simulink model "esempio1S"  (R2021a)
settings: Solver=VariableStepAuto  StartTime=0.0  StopTime=10.0  RelTol=1e-3
values from neighbouring files (symbols this model uses):
  A = [0 1; 0 -2]    [esempio.m]    (also in esempio1.m = [-2 1; -2 0]; esempio2.m = [0 1; 2 1])
  B = [ 0; 1]    [esempio.m]    (also in esempio1.m = [0; 1]; esempio2.m = [0; 1])
  C = eye(2)    [esempio.m]    (also in esempio1.m; esempio2.m)
  D = zeros(2,1)    [esempio.m]    (also in esempio1.m; esempio2.m)
  K = place(A, B, P)    [esempio.m]    (also in esempio1.m = acker(A, B, P); esempio2.m)
  x0 = [0;0]    [esempio1.m]
settings Model: Creator=itama  LastModifiedBy=itama
settings SolverCC: AlgebraicLoopSolver=TrustRegion
settings DebuggingCC: SFMachineParentedDataDiag=warning

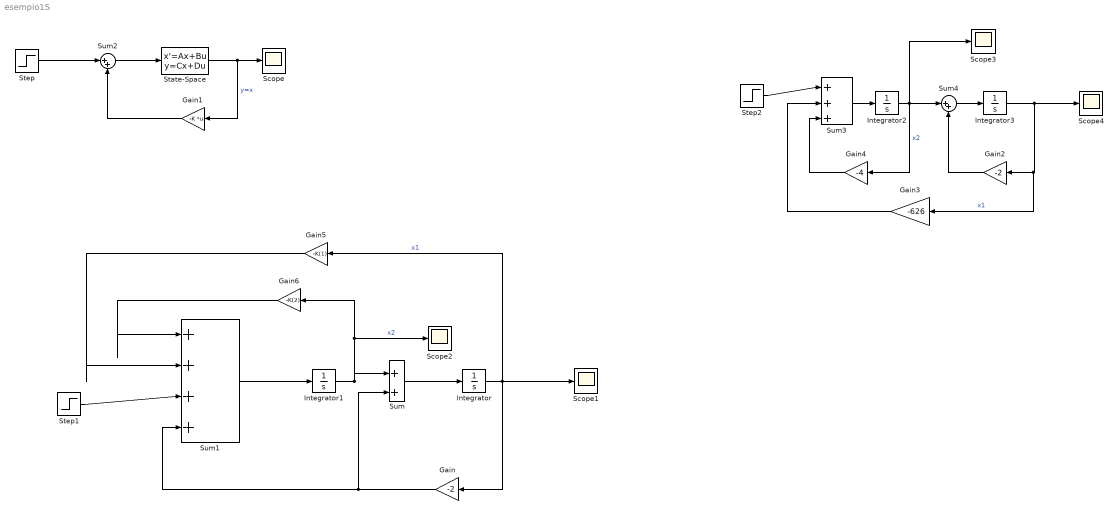
== system esempio1S ==
  Gain : Gain  Gain=-2
  Gain1 : Gain  Gain=-K  Multiplication=Matrix(K*u)
  Gain2 : Gain  Gain=-2
  Gain3 : Gain  Gain=-626
  Gain4 : Gain  Gain=-4
  Gain5 : Gain  Gain=-K(1)
  Gain6 : Gain  Gain=-K(2)
  Integrator{,1..3} (4 alike) : Integrator
  Scope{,1..4} (5 alike) : Scope
  State-Space : StateSpace  A=A  B=B  C=C  D=D  InitialCondition=x0
  Step : Step  SampleTime=0
  Step1 : Step  SampleTime=0
  Step2 : Step  SampleTime=0
  Sum : Sum  Inputs=|++
  Sum1 : Sum  Inputs=|++++
  Sum2 : Sum  Inputs=|++
  Sum3 : Sum  Inputs=|+++
  Sum4 : Sum  Inputs=|++
  wires:
  State-Space/1 -> Gain1/1, Scope/1  "y=x"
  Integrator/1 -> Gain5/1, Gain/1, Scope1/1  "x1"
  Integrator1/1 -> Sum/1, Gain6/1, Scope2/1  "x2"
  Gain/1 -> Sum1/4, Sum/2
  Sum/1 -> Integrator/1
  Sum1/1 -> Integrator1/1
  Gain1/1 -> Sum2/2
  Integrator3/1 -> Gain3/1, Gain2/1, Scope4/1  "x1"
  Sum3/1 -> Integrator2/1
  Step2/1 -> Sum3/1
  Gain2/1 -> Sum4/2
  Integrator2/1 -> Gain4/1, Scope3/1, Sum4/1  "x2"
  Gain3/1 -> Sum3/2
  Gain4/1 -> Sum3/3
  Sum4/1 -> Integrator3/1
  Sum2/1 -> State-Space/1
  Step/1 -> Sum2/1
  Step1/1 -> Sum1/3
  Gain5/1 -> Sum1/2
  Gain6/1 -> Sum1/1
